simulink model "SMDFR"  (R2024b)
settings: Solver=ode15s  StartTime=1  StopTime=1200  FixedStep=0.01  RelTol=1e-3
model workspace (MAT data in the model file):
  ACS_lambda = 0.000161129786201
  A_cucl = 134.446
  A_cucl2 = 134.446
  A_cuocl = 213.991
  A_d = 217.647058824
  A_fw = [13.6 90 13.6]
  A_h = 217.647058824
  A_h2 = 217.647058824
  A_h20 = 18.015
  A_hcl = 36.458
  A_o = 32
  A_sg = 370
  A_wc = [10.9 103 10.9]
  C_c = 140.2
  C_cucl = 0.71
  C_cuocl = 1
  C_dst = 1996000
  C_h20 = 4.48
  C_hcl = 0.8
  C_hst = 1996000
  C_i0 = [429000000000000; 4.15e+15; 3.83e+15; 1.16e+16; 5.7e+15; 1.53e+15]
  C_o = 0.918
  Ce_i0 = [701000000000000; 5.88e+15; 3.36e+15; 5.09e+15; 820000000000000; 39600000000000]
  Cr = 0.00113148387097
  Cr_m = 8.769
  Cr_m_red = 4.3845
  Cr_red = 0.000565741935484
  D = 0.16
  DPB_lambda = 0.01
  EPB_lambda = 0.01
  E_d = 5
  E_e = 5
  E_h = 5
  E_hte = 5
  G_cucl = 44.778
  G_cucl2 = 44.778
  G_cuocl = 35.6355
  G_h2 = 32
  G_h20 = 10
  G_h20i = 10
  G_h20o = 7
  G_hcl = 12.1426
  G_o = 2.66
  G_s = 27000
  H_valve = 1
  Heat = [18744000 5970000 16956000]
  IPB_lambda = 0.01
  K_d = 500
  K_h = 500
  L = 6
  LOCA1 = 0
  LOCA2 = 0
  LOCA3 = 0
  LOCA4 = 0
  LOCA_p = 0.000161129786201
  LOCA_time = 300
  LOCA_times = [408 453 64 457 317 49 140 274 479 483 79 486 ... (4000 elements, 1000x4)]
  LOPC = 0
  LOPC_p = 0.1
  LOPC_times = [214 478 363 291 271 353 3 392 464 5 413 384 ... (1000 elements, 1000x1)]
  L_ACS = 0.01
  Lambda = 1.05e-06
  M_c = [219.9 7705 219.9]
  M_cucl0 = 44.778
  M_cucl20 = 44.778
  M_f = [307.7 1164 307.7]
  M_h20 = 8
  M_hcl0 = 12.1426
  M_w = [39.3 311 39.3]
  N = 1000
  N_0 = 15000000000000
  Nodes = 3
  P_0 = 100000000
  P_decomposition = 160
  P_hydro = 167
  Pb_acs : object (value not decoded)
  Pb_pipes : object (value not decoded)
  Pi_0 = [0.158 0.6899 0.152]
  Power_lambda = 0.01
  RPB_lambda = 0.01
  T_fw = 300
  T_hpi = 100
  T_st = 900
  Tbar_c0 = 1060
  Tbar_f0 = 1288
  Tc_in = 973
  Tin_c = 973
  Tin_f = 1300
  Tout_c = 1100
  Tout_f = 1300
  V_c = 160
  V_d = 160
  V_dst = 100
  V_h = 160
  V_h2 = 160
  V_hst = 100
  V_s = 100
  V_sg = 100
  age = 0
  ages = [0 50]
  alfa_c = -8.28e-06
  alfa_f = -0.000208
  alpha = 0.9926
  alpha_1 = 1
  alpha_2 = 1
  alpha_3 = 1
  alpha_4 = 1
  beta = 0.00302
  beta_i = [7.91e-05 0.000703 0.000504 0.00117 0.000457 0.00011]
  c_pc = [140.2 140.2 140.2]
  c_pf = [400 400 400]
  c_pw = [690 690 690]
  coolpipes = [2166 2166 0]
  d_c = 10187.40024
  d_dst = 3.14
  d_hst = 3.14
  d_st = 6.123
  diesel_lambda = 0.01
  eta = 0.4
  fail_threshold = 1244
  file = 'SMDFR_Parameters'
  fuelpipes = 1027
  h_dpo = 6801000
  h_fw = [6546 4305.1 7629.5]
  h_fw_st = 4386450
  h_hpo = 7159680
  h_in = 7000
  h_out = 1000
  h_st_in = 4386450
  h_wc = [27405.4 13833.4 32177.3]
  i = 1
  j = 1
  k_d = 2.7187
  k_e = 2.7187
  k_h = 0.005
  k_hte = 2.7187
  k_sg = 500
  lambda_c = 0.184
  lambda_e = 0.1
  lambda_i = [0.0127 0.03 0.11 0.319 1.18 7.02]
  leakage = 6.5
  mdot_c = [5550.5 5550.5 5550.5]
  mdot_c_value = 5550.5
  mdot_f = [327.7 327.7 327.7]
  mdot_f_value = 327.7
  model = 'SMDFR'
  mu = 50.9722799688
  mu_f = -20.9722799688
  mu_o = 30
  n = 0.45
  nsim = 1
  p_h20 = 40
  phi_tot = 3.61e+21
  rho = 7750
  rho_0 = 0.00111
  rhoex_value = 0
  sigma = 625
  sigma_c = 5
  sigma_f = 5.83095189485
  sigma_o = 3
  step = 0.1
  t = 0.008
  tau_c = 5.43
  tau_e = 10
  tsim = 500
  v_rec = 4.16e-09
values from neighbouring files (symbols this model uses):
  ACS1_flow = 25    [Only_Inputs.m]    (also in Simulation_model.m; Simulation_model_complete.m; Simulation_model_hydrogen.m; Simulation_model_hydrogen_parallel.m)
  ACS1_response_time = randi(t_max_r_ACS-t_min_r_ACS)+t_min_r_ACS    [Failure_model.m]    (also in Failure_model_outputs.mat = 36; Only_Inputs.m = ACS1_response_time(indexes))
  ACS2_flow = 25    [Only_Inputs.m]    (also in Simulation_model.m; Simulation_model_complete.m; Simulation_model_hydrogen.m; Simulation_model_hydrogen_parallel.m)
  ACS2_response_time = randi(t_max_r_ACS-t_min_r_ACS)+t_min_r_ACS    [Failure_model.m]    (also in Failure_model_outputs.mat = 49; Only_Inputs.m = ACS2_response_time(indexes); Simulation_model_hydrogen_parallel.m = 0)
  ACS3_flow = 25    [Only_Inputs.m]    (also in Simulation_model.m; Simulation_model_complete.m; Simulation_model_hydrogen.m; Simulation_model_hydrogen_parallel.m)
  ACS3_response_time = randi(t_max_r_ACS-t_min_r_ACS)+t_min_r_ACS    [Failure_model.m]    (also in Failure_model_outputs.mat = 62; Only_Inputs.m = ACS3_response_time(indexes); Simulation_model_hydrogen_parallel.m = 0)
  ACS4_flow = 25    [Only_Inputs.m]    (also in Simulation_model.m; Simulation_model_complete.m; Simulation_model_hydrogen.m; Simulation_model_hydrogen_parallel.m)
  ACS4_response_time = randi(t_max_r_ACS-t_min_r_ACS)+t_min_r_ACS    [Failure_model.m]    (also in Failure_model_outputs.mat = 57; Only_Inputs.m = ACS4_response_time(indexes); Simulation_model_hydrogen_parallel.m = 0)
  ACS_1 = 821    [Failure_model_outputs.mat]    (also in Failure_sim.m = ACS_times(1); Only_Inputs.m = ACS_1(indexes))
  ACS_2 = 1010    [Failure_model_outputs.mat]    (also in Failure_sim.m = ACS_times(2); Only_Inputs.m = ACS_2(indexes); Simulation_model_hydrogen_parallel.m = 1)
  ACS_3 = 926    [Failure_model_outputs.mat]    (also in Failure_sim.m = ACS_times(3); Only_Inputs.m = ACS_3(indexes); Simulation_model_hydrogen_parallel.m = 1)
  ACS_4 = 80    [Failure_model_outputs.mat]    (also in Failure_sim.m = ACS_times(4); Only_Inputs.m = ACS_4(indexes); Simulation_model_hydrogen_parallel.m = 1)
  All_Outputs = 1    [Only_Inputs.m]    (also in Simulation_model.m = 0; Simulation_model_complete.m = 0; Simulation_model_hydrogen.m = 0; Simulation_model_hydrogen_parallel.m = 0)
  EDG1_response_time = randi(t_max_r_EDG-t_min_r_EDG)+t_min_r_EDG    [Failure_model.m]    (also in Failure_model_outputs.mat = 170; Only_Inputs.m = EDG1_response_time(indexes))
  EDG2_response_time = randi(t_max_r_EDG-t_min_r_EDG)+t_min_r_EDG    [Failure_model.m]    (also in Failure_model_outputs.mat = 133; Only_Inputs.m = EDG2_response_time(indexes); Simulation_model_hydrogen_parallel.m = 0)
  EDG_1 = 567    [Failure_model_outputs.mat]    (also in Only_Inputs.m = EDG_1(indexes))
  EDG_2 = 323    [Failure_model_outputs.mat]    (also in Only_Inputs.m = EDG_2(indexes); Simulation_model_hydrogen_parallel.m = 1)
  LOCA1_time = 1200    [Failure_model_outputs.mat]    (also in Failure_sim.m = loca_times(1); Only_Inputs.m = LOCA1_time(indexes))
  LOCA2_time = 1200    [Failure_model_outputs.mat]    (also in Failure_sim.m = loca_times(2); Only_Inputs.m = LOCA2_time(indexes); Simulation_model_hydrogen_parallel.m)
  LOCA3_time = 39    [Failure_model_outputs.mat]    (also in Failure_sim.m = loca_times(3); Only_Inputs.m = LOCA3_time(indexes); Simulation_model_hydrogen_parallel.m = 1200)
  LOCA4_time = 18    [Failure_model_outputs.mat]    (also in Failure_sim.m = loca_times(4); Only_Inputs.m = LOCA4_time(indexes); Simulation_model_hydrogen_parallel.m = 1200)
  MSLB1 = 1200    [Failure_model_outputs.mat]    (also in Failure_sim.m = fix(randsample(x_loca, 1, true, lognorm_pdf)); Only_Inputs.m = MSLB1(indexes))
  MSLB2 = 1200    [Failure_model_outputs.mat]    (also in Failure_sim.m = fix(randsample(x_loca, 1, true, lognorm_pdf)); Only_Inputs.m = MSLB2(indexes); Simulation_model_hydrogen_parallel.m = 0)
  MSLB3 = 1200    [Failure_model_outputs.mat]    (also in Failure_sim.m = fix(randsample(x_loca, 1, true, lognorm_pdf)); Only_Inputs.m = MSLB3(indexes); Simulation_model_hydrogen_parallel.m = 0)
  MSLB4 = 1200    [Failure_model_outputs.mat]    (also in Failure_sim.m = fix(randsample(x_loca, 1, true, lognorm_pdf)); Only_Inputs.m = MSLB4(indexes); Simulation_model_hydrogen_parallel.m = 0)
  PDP11 = 1200    [Failure_model_outputs.mat]    (also in Failure_sim.m = pdp_times(1); Only_Inputs.m = PDP11(indexes))
  PDP11_response_time = randi(t_max_r_EDG-t_min_r_EDG)+t_min_r_EDG    [Failure_model.m]    (also in Failure_model_outputs.mat = 136; Only_Inputs.m = PDP11_response_time(indexes))
  PDP12 = 1200    [Failure_model_outputs.mat]    (also in Failure_sim.m = pdp_times(2); Only_Inputs.m = PDP12(indexes); Simulation_model_hydrogen_parallel.m = 0)
  PDP12_response_time = randi(t_max_r_EDG-t_min_r_EDG)+t_min_r_EDG    [Failure_model.m]    (also in Failure_model_outputs.mat = 119; Only_Inputs.m = PDP12_response_time(indexes); Simulation_model_hydrogen_parallel.m = 0)
  PDP21 = 1200    [Failure_model_outputs.mat]    (also in Failure_sim.m = pdp_times(3); Only_Inputs.m = PDP21(indexes); Simulation_model_hydrogen_parallel.m = 0)
  PDP21_response_time = randi(t_max_r_EDG-t_min_r_EDG)+t_min_r_EDG    [Failure_model.m]    (also in Failure_model_outputs.mat = 17; Only_Inputs.m = PDP21_response_time(indexes); Simulation_model_hydrogen_parallel.m = 0)
  PDP22 = 1200    [Failure_model_outputs.mat]    (also in Failure_sim.m = pdp_times(4); Only_Inputs.m = PDP22(indexes); Simulation_model_hydrogen_parallel.m = 0)
  PDP22_response_time = randi(t_max_r_EDG-t_min_r_EDG)+t_min_r_EDG    [Failure_model.m]    (also in Failure_model_outputs.mat = 120; Only_Inputs.m = PDP22_response_time(indexes); Simulation_model_hydrogen_parallel.m = 0)
  PDP31 = 1200    [Failure_model_outputs.mat]    (also in Failure_sim.m = pdp_times(5); Only_Inputs.m = PDP31(indexes); Simulation_model_hydrogen_parallel.m = 0)
  PDP31_response_time = randi(t_max_r_EDG-t_min_r_EDG)+t_min_r_EDG    [Failure_model.m]    (also in Failure_model_outputs.mat = 65; Only_Inputs.m = PDP31_response_time(indexes); Simulation_model_hydrogen_parallel.m = 0)
  PDP32 = 1200    [Failure_model_outputs.mat]    (also in Failure_sim.m = pdp_times(6); Only_Inputs.m = PDP32(indexes); Simulation_model_hydrogen_parallel.m = 0)
  PDP32_response_time = randi(t_max_r_EDG-t_min_r_EDG)+t_min_r_EDG    [Failure_model.m]    (also in Failure_model_outputs.mat = 28; Only_Inputs.m = PDP32_response_time(indexes); Simulation_model_hydrogen_parallel.m = 0)
  PDP41 = 1200    [Failure_model_outputs.mat]    (also in Failure_sim.m = pdp_times(7); Only_Inputs.m = PDP41(indexes); Simulation_model_hydrogen_parallel.m = 0)
  PDP41_response_time = randi(t_max_r_EDG-t_min_r_EDG)+t_min_r_EDG    [Failure_model.m]    (also in Failure_model_outputs.mat = 24; Only_Inputs.m = PDP41_response_time(indexes); Simulation_model_hydrogen_parallel.m = 0)
  PDP42 = 1200    [Failure_model_outputs.mat]    (also in Failure_sim.m = pdp_times(8); Only_Inputs.m = PDP42(indexes); Simulation_model_hydrogen_parallel.m = 0)
  PDP42_response_time = randi(t_max_r_EDG-t_min_r_EDG)+t_min_r_EDG    [Failure_model.m]    (also in Failure_model_outputs.mat = 164; Only_Inputs.m = PDP42_response_time(indexes); Simulation_model_hydrogen_parallel.m = 0)
  Power = 1200    [Failure_model_outputs.mat]    (also in Failure_sim.m = fix(randsample(x_loca, 1, true, lognorm_pdf)); Only_Inputs.m = Power(indexes))
libraries: SMDFR_lib x8
(part 2 of 2)

== matlab function SMDFR/MATLAB Function14 ==
  data: t input; PDP1_fail output; MSLB3 parameter; PDP31_response_time parameter; PDP31 parameter; EDG input
function PDP1_fail = fcn(t,MSLB3, PDP31_response_time, PDP31, EDG)

if ((t<PDP31 || EDG) && t>(MSLB3+PDP31_response_time)) 
    PDP1_fail=0;
else
    PDP1_fail=1;
end

== matlab function SMDFR/MATLAB Function15 ==
  data: t input; PDP2_fail output; MSLB3 parameter; PDP32_response_time parameter; PDP32 parameter; EDG input
function PDP2_fail = fcn(t,MSLB3, PDP32_response_time, PDP32, EDG)

if ((t<PDP32 || EDG) && t>(MSLB3+PDP32_response_time)) 
    PDP2_fail=0;
else
    PDP2_fail=1;
end

== matlab function SMDFR/MATLAB Function2 ==
  data: ACS input; y output; time input
function y = fcn(ACS,time)

if time > ACS
    y=0;
else
    y=1;
end

== matlab function SMDFR/MATLAB Function1 ==
  data: ACS input; y output; time input
function y = fcn(ACS,time)

if time > ACS
    y=0;
else
    y=1;
end

== matlab function SMDFR/MATLAB Function3 ==
  data: ACS input; y output; time input
function y = fcn(ACS,time)

if time > ACS
    y=0;
else
    y=1;
end

== matlab function SMDFR/MATLAB Function4 ==
  data: ACS input; y output; time input
function y= fcn(ACS,time)

if time > ACS
    y=0;
else
    y=1;
end

== matlab function SMDFR/MATLAB Function5 ==
  data: EDG input; LOP input; response_time input; EDG_working output; time input
function EDG_working = fcn(EDG,LOP, response_time, time)

if time > EDG
    EDG_working=0;
else
    if (time-LOP)>response_time
        EDG_working=1;
    else
        EDG_working=0;
    end
end

== matlab function SMDFR/MATLAB Function6 ==
  data: EDG input; LOP input; response_time input; EDG_working output; time input
function EDG_working = fcn(EDG,LOP, response_time, time)

if time > EDG
    EDG_working=0;
else
    if (time-LOP)>response_time
        EDG_working=1;
    else
        EDG_working=0;
    end
end

== matlab function SMDFR/MATLAB Function7 ==
  data: LOP input; Power_out output; time input
function Power_out = fcn(LOP,time)

if time > LOP
    Power_out=0;
else
    Power_out=1;
end
